simulink model "gm_Moving_Average_sim"  (R2025a)
settings: Solver=VariableStepAuto  StartTime=0.0  StopTime=20  RelTol=1e-3
libraries: hdlmdlgenlib x1, simulink x1
settings Model: Creator=Luiz  LastModifiedBy=Luiz
settings OptimizationCC: BlockReduction=off  ConditionallyExecuteInputs=off  DefaultParameterBehavior=Inlined
settings DebuggingCC: AlgebraicLoopMsg=error  InheritedTsInSrcMsg=none  SingleTaskRateTransMsg=error
settings HardwareCC: ProdBitPerPointer=32.0  ProdBitPerSizeT=32.0  ProdBitPerPtrDiffT=32.0  ProdLargestAtomicFloat=None  ProdIntDivRoundTo=Undefined  ProdEndianess=Unspecified  ProdWordSize=32.0  ProdHWDeviceType=ASIC/FPGA->ASIC/FPGA  TargetBitPerPointer=64.0  TargetBitPerSizeT=64.0  TargetBitPerPtrDiffT=64.0  TargetLongLongMode=on  TargetIntDivRoundTo=Zero  TargetEndianess=LittleEndian  TargetWordSize=64.0  TargetHWDeviceType=Custom Processor->MATLAB Host Computer  ProdEqTarget=off

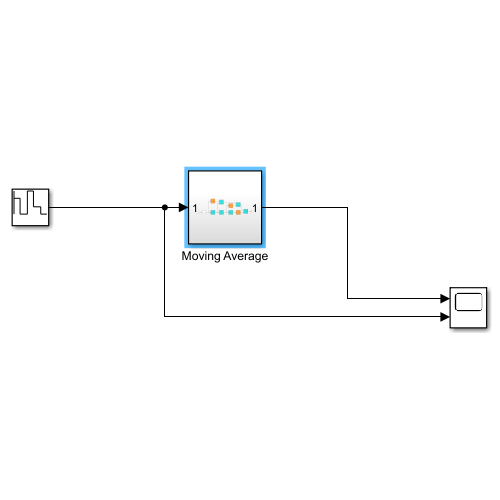
[thumbnail: Simulink's stored preview of the top-level diagram]
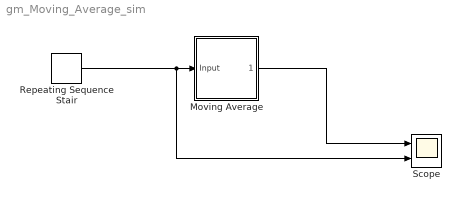
== system gm_Moving_Average_sim ==
  Moving Average : Subsystem
  Repeating Sequence Stair : simulink/Sources/Repeating Sequence Stair  OutValues=[3 1 4 2 1].'  tsamp=-1  OutMin=[]  OutMax=[]  OutDataTypeStr=double  OutputDataTypeScalingMode=double  OutDataType=fixdt(0,8)  ConRadixGroup=Best Precision: Vector-wise  OutScaling=2^-12
      settings: LibrarySourceBlock=|
      | hdlsllib/Sources/Repeating
      | Sequence
      | Stair
  Scope : Scope  NumInputPorts=2
      settings: ActiveDisplayYMinimum=-630.21833750871519  ActiveDisplayYMaximum=398.16860392885332  DataLoggingVariableName=ScopeData2  DataLoggingSaveFormat=Array
  wires:
  Moving Average/1(Output) -> Scope/1
  Repeating Sequence Stair/1 -> Moving Average/1(Input), Scope/2

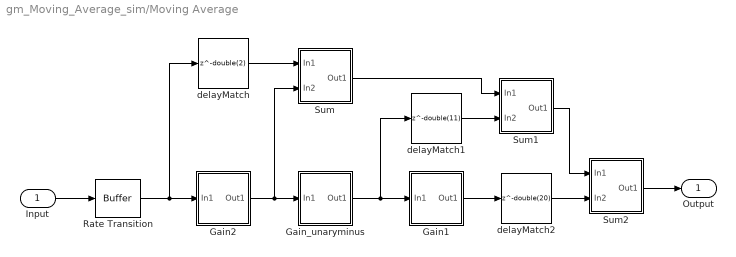
== system gm_Moving_Average_sim/Moving Average ==
  Input : Inport  OutDataTypeStr=double  PortDimensions=1  SampleTime=0.0001
  Gain1 : Subsystem
      mask Display: disp('NFP\ngain_pow2');
  Gain2 : Subsystem
      mask Display: disp('NFP\ngain_pow2');
  Gain_unaryminus : Subsystem
      mask Display: disp('NFP\numinus');
  Rate Transition : hdlmdlgenlib/Buffer
  Sum : Subsystem
      mask Display: disp('NFP\nadd');
  Sum1 : Subsystem
      mask Display: disp('NFP\nadd');
  Sum2 : Subsystem
      mask Display: disp('NFP\nadd');
  delayMatch : Delay  DelayLength=double(2)  InitialCondition=0  SampleTime=0.0001
  delayMatch1 : Delay  DelayLength=double(11)  InitialCondition=0  SampleTime=0.0001
  delayMatch2 : Delay  DelayLength=double(20)  InitialCondition=0  SampleTime=0.0001
  Output : Outport  OutDataTypeStr=double  SampleTime=0.0001  VectorParamsAs1DForOutWhenUnconnected=off
  wires:
  Gain1/1(Out1) -> delayMatch2/1
  delayMatch/1 -> Sum/1(In1)
  Input/1 -> Rate Transition/1
  Gain_unaryminus/1(Out1) -> delayMatch1/1, Gain1/1(In1)
  Rate Transition/1 -> Gain2/1(In1), delayMatch/1
  Gain2/1(Out1) -> Sum/2(In2), Gain_unaryminus/1(In1)
  Sum/1(Out1) -> Sum1/1(In1)
  delayMatch1/1 -> Sum1/2(In2)
  Sum1/1(Out1) -> Sum2/1(In1)
  delayMatch2/1 -> Sum2/2(In2)
  Sum2/1(Out1) -> Output/1

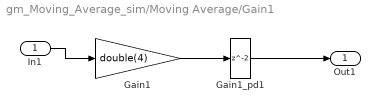
== system gm_Moving_Average_sim/Moving Average/Gain1 ==
  In1 : Inport
  Gain1 : Gain  Gain=double(4)
  Gain1_pd1 : Delay
  Out1 : Outport
  wires:
  In1/1 -> Gain1/1
  Gain1/1 -> Gain1_pd1/1
  Gain1_pd1/1 -> Out1/1

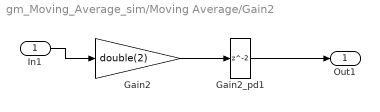
== system gm_Moving_Average_sim/Moving Average/Gain2 ==
  In1 : Inport
  Gain2 : Gain  Gain=double(2)
  Gain2_pd1 : Delay
  Out1 : Outport
  wires:
  In1/1 -> Gain2/1
  Gain2/1 -> Gain2_pd1/1
  Gain2_pd1/1 -> Out1/1

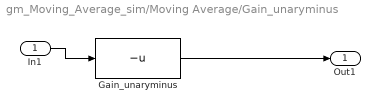
== system gm_Moving_Average_sim/Moving Average/Gain_unaryminus ==
  In1 : Inport
  Gain_unaryminus : UnaryMinus  SampleTime=0.0001
  Out1 : Outport
  wires:
  In1/1 -> Gain_unaryminus/1
  Gain_unaryminus/1 -> Out1/1

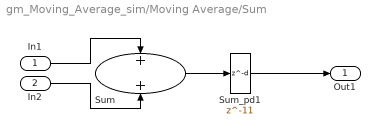
== system gm_Moving_Average_sim/Moving Average/Sum ==
  In1 : Inport
  In2 : Inport  Port=2
  Sum : Sum  OutDataTypeStr=double  SampleTime=0.0001
  Sum_pd1 : Delay  DelayLength=11
  Out1 : Outport
  wires:
  In1/1 -> Sum/1
  In2/1 -> Sum/2
  Sum/1 -> Sum_pd1/1
  Sum_pd1/1 -> Out1/1

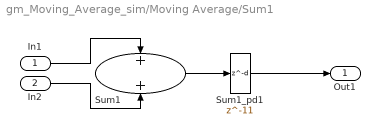
== system gm_Moving_Average_sim/Moving Average/Sum1 ==
  In1 : Inport
  In2 : Inport  Port=2
  Sum1 : Sum  OutDataTypeStr=double  SampleTime=0.0001
  Sum1_pd1 : Delay  DelayLength=11
  Out1 : Outport
  wires:
  In1/1 -> Sum1/1
  In2/1 -> Sum1/2
  Sum1/1 -> Sum1_pd1/1
  Sum1_pd1/1 -> Out1/1

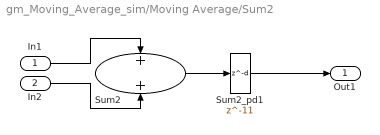
== system gm_Moving_Average_sim/Moving Average/Sum2 ==
  In1 : Inport
  In2 : Inport  Port=2
  Sum2 : Sum  OutDataTypeStr=double  SampleTime=0.0001
  Sum2_pd1 : Delay  DelayLength=11
  Out1 : Outport
  wires:
  In1/1 -> Sum2/1
  In2/1 -> Sum2/2
  Sum2/1 -> Sum2_pd1/1
  Sum2_pd1/1 -> Out1/1
